simulink model "parts"  (R2021b)
settings: Solver=ode15s  StartTime=0.0  StopTime=t_f  MaxStep=max_step_size  RelTol=1e-3
values from neighbouring files (symbols this model uses):
  cont_param_10 = in    [double_pendulum.m]    (also in optimize_10_SMC_single_first_explicit.m = cont_param_10_surrogateopt)
  cont_param_11 = in    [double_pendulum.m]    (also in optimize_11_SMC_single_first_implicit.m = cont_param_11_surrogateopt)
  cont_param_12 = in    [double_pendulum.m]    (also in optimize_12_SMC_single_last_explicit.m = cont_param_12_surrogateopt)
  cont_param_13 = in    [double_pendulum.m]    (also in optimize_13_SMC_single_last_implicit.m = cont_param_13_surrogateopt)
  cont_param_14 = in    [double_pendulum.m]    (also in optimize_14_SMC_double_explicit.m = cont_param_14_surrogateopt)
  cont_param_15 = in    [double_pendulum.m]    (also in optimize_15_SMC_double_implicit.m = cont_param_15_surrogateopt)
  cont_param_16 = in    [double_pendulum.m]
  cont_param_17 = in    [double_pendulum.m]
  cont_param_18 = in    [double_pendulum.m]
  cont_param_19 = in    [double_pendulum.m]
  cont_param_4 = in    [double_pendulum.m]
  cont_param_5 = in    [double_pendulum.m]
  cont_param_6 = in    [double_pendulum.m]
  cont_param_7 = in    [double_pendulum.m]
  cont_param_8 = in    [double_pendulum.m]
  cont_param_9 = in    [double_pendulum.m]
  h = 1e-5    (= 1e-05)    [Conference_paper.m]    (also in Latest.m)
  m = 10    [Conference_paper.m]    (also in Latest.m = 100; control_8_collocated_PD_tracking.m = load_mass+hook_mass+cable_mass_total)
  method_select = Method    [main_run.m]    (also in modify_tracking.m = 3)
  N = floor(t_f / h)    [control_2_zero_vibration.m]    (also in control_3_ZVD.m; modify_tracking.m = 3)
  s = c1*(x-xd)+c2*(v-vd)+c3*theta_dot_1+c4*theta_1    [control_10_SMC_single_first_explicit.m]    (also in control_11_SMC_single_first_implicit.m = c1*(x-xd)+c2*(v-vd)+c3*theta_dot+c4*theta; control_12_SMC_single_last_explicit.m = c1*(x-xd)+c2*(v-vd)+c3*theta_dot_2+c4*theta_2; control_13_SMC_single_last_implicit.m = c1*(x-xd)+c2*(v-vd)+c3*theta_dot+c4*theta; control_14_SMC_double_explicit.m = (v-vd)+lambda*(x-xd)+alpha*theta_1+beta*theta_2)
  X = ex+lambda*sin(theta)    [control_16_PD_energy_first.m]    (also in control_17_PD_energy_last.m)
  Z = cont_param_8(4)    [control_8_collocated_PD_tracking.m]
undefined symbols (not defined in the file or in its folder): a_d_full, all_initial_sway, c_actuator, cable_eact_piece, cable_length, cable_mass_total, cart_disturbance_amp, cart_mass, delay_time, first_link_sway, hook_mass, last_piece_length, load_disturbance_amp, number_of_pendulums, payload_mass, sat_const, t_f, total_mass, traj_number, Y
libraries: sm_lib x72, nesl_utility x47, commchan3 x4
(part 2 of 2)

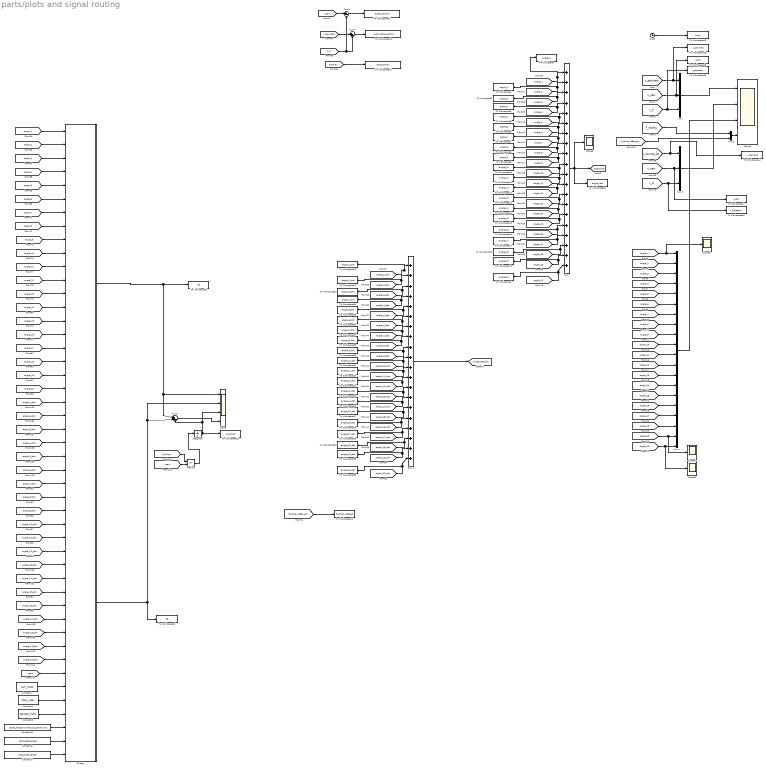
== system parts/plots and signal routing ==
  Clock : Clock
  Constant : Constant  Value=cart_mass
  Constant1 : Constant  Value=hook_mass
  Constant11 : Constant  Value=cable_length/number_of_pendulums
  Constant2 : Constant  Value=payload_mass
  Constant3 : Constant  Value=cable_eact_piece
  Constant4 : Constant  Value=last_piece_length
  Energy : MATLAB Function  TreatAsAtomicUnit=on
  Integrator : Integrator
  Mux : Mux  Inputs=3
  Mux1 : Mux  Inputs=20
  Mux2 : Mux  Inputs=3
  Mux3 : Mux  Inputs=2
  Product : Product
  Scope : Scope  NumInputPorts=4
  Scope1 : Scope  NumInputPorts=4
  Scope{3..6} (4 alike) : Scope
  Sum : Sum  Inputs=|++++++++++++++++++++
  Sum1 : Sum  Inputs=|++++++++++++++++++++
  Sum2 : Sum  Inputs=|+-
  Sum3 : Sum  Inputs=|+-
  Sum4 : Sum  Inputs=|++-
  To Workspace : ToWorkspace  VariableName=angle_1  SampleTime=-1
  To Workspace1 : ToWorkspace  VariableName=angle_2  SampleTime=-1
  To Workspace10 : ToWorkspace  VariableName=angle_10  SampleTime=-1
  To Workspace11 : ToWorkspace  VariableName=angle_11  SampleTime=-1
  To Workspace12 : ToWorkspace  VariableName=angle_12  SampleTime=-1
  To Workspace13 : ToWorkspace  VariableName=angle_13  SampleTime=-1
  To Workspace14 : ToWorkspace  VariableName=angle_14  SampleTime=-1
  To Workspace15 : ToWorkspace  VariableName=angle_15  SampleTime=-1
  To Workspace16 : ToWorkspace  VariableName=angle_16  SampleTime=-1
  To Workspace17 : ToWorkspace  VariableName=angle_17  SampleTime=-1
  To Workspace18 : ToWorkspace  VariableName=angle_18  SampleTime=-1
  To Workspace19 : ToWorkspace  VariableName=angle_19  SampleTime=-1
  To Workspace2 : ToWorkspace  VariableName=angle_3  SampleTime=-1
  To Workspace20 : ToWorkspace  VariableName=angle_1_dot  SampleTime=-1
  To Workspace21 : ToWorkspace  VariableName=angle_2_dot  SampleTime=-1
  To Workspace22 : ToWorkspace  VariableName=angle_10_dot  SampleTime=-1
  To Workspace23 : ToWorkspace  VariableName=angle_11_dot  SampleTime=-1
  To Workspace24 : ToWorkspace  VariableName=angle_12_dot  SampleTime=-1
  To Workspace25 : ToWorkspace  VariableName=angle_13_dot  SampleTime=-1
  To Workspace26 : ToWorkspace  VariableName=angle_14_dot  SampleTime=-1
  To Workspace27 : ToWorkspace  VariableName=angle_15_dot  SampleTime=-1
  To Workspace28 : ToWorkspace  VariableName=angle_16_dot  SampleTime=-1
  To Workspace29 : ToWorkspace  VariableName=angle_17_dot  SampleTime=-1
  To Workspace3 : ToWorkspace  VariableName=angle_20  SampleTime=-1
  To Workspace30 : ToWorkspace  VariableName=angle_18_dot  SampleTime=-1
  To Workspace31 : ToWorkspace  VariableName=angle_19_dot  SampleTime=-1
  To Workspace32 : ToWorkspace  VariableName=angle_3_dot  SampleTime=-1
  To Workspace33 : ToWorkspace  VariableName=angle_20_dot  SampleTime=-1
  To Workspace34 : ToWorkspace  VariableName=angle_4_dot  SampleTime=-1
  To Workspace35 : ToWorkspace  VariableName=angle_5_dot  SampleTime=-1
  To Workspace36 : ToWorkspace  VariableName=angle_6_dot  SampleTime=-1
  To Workspace37 : ToWorkspace  VariableName=angle_7_dot  SampleTime=-1
  To Workspace38 : ToWorkspace  VariableName=angle_8_dot  SampleTime=-1
  To Workspace39 : ToWorkspace  VariableName=angle_9_dot  SampleTime=-1
  To Workspace4 : ToWorkspace  VariableName=angle_4  SampleTime=-1
  To Workspace40 : ToWorkspace  VariableName=e_payload_position  SampleTime=-1
  To Workspace41 : ToWorkspace  VariableName=Force_trolley  SampleTime=-1
  To Workspace42 : ToWorkspace  VariableName=e_cart_position  SampleTime=-1
  To Workspace43 : ToWorkspace  VariableName=x_payload  SampleTime=-1
  To Workspace44 : ToWorkspace  VariableName=v_payload  SampleTime=-1
  To Workspace45 : ToWorkspace  VariableName=x_cart  SampleTime=-1
  To Workspace46 : ToWorkspace  VariableName=x_trajectory  SampleTime=-1
  To Workspace47 : ToWorkspace  VariableName=v_cart  SampleTime=-1
  To Workspace48 : ToWorkspace  VariableName=v_trajectory  SampleTime=-1
  To Workspace49 : ToWorkspace  VariableName=time  SampleTime=-1
  To Workspace5 : ToWorkspace  VariableName=angle_5  SampleTime=-1
  To Workspace50 : ToWorkspace  VariableName=angle_last  SampleTime=-1
  To Workspace51 : ToWorkspace  VariableName=KE  SampleTime=-1
  To Workspace52 : ToWorkspace  VariableName=PE  SampleTime=-1
  To Workspace53 : ToWorkspace  VariableName=supplied  SampleTime=-1
  To Workspace54 : ToWorkspace  VariableName=F_trolley_filtered  SampleTime=-1
  To Workspace6 : ToWorkspace  VariableName=angle_6  SampleTime=-1
  To Workspace7 : ToWorkspace  VariableName=angle_7  SampleTime=-1
  To Workspace8 : ToWorkspace  VariableName=angle_8  SampleTime=-1
  To Workspace9 : ToWorkspace  VariableName=angle_9  SampleTime=-1
  tag scope: angle_last=global, angle_last_dot=global
  wires:
  Mux/1 -> Scope1/1
  [x_payload] -> To Workspace43/1, Mux/1  "x_payload"
  [x_cart] -> To Workspace45/1, Mux/2  "x_cart"
  [x_d] -> To Workspace46/1, Mux/3  "x_trajectory"
  Mux1/1 -> Scope1/3
  [angle_1] -> Scope3/1, Mux1/1  "Angle 1"
  [angle_2] -> Mux1/2  "Angle 2"
  [angle_3] -> Mux1/3  "Angle 3"
  [angle_4] -> Mux1/4  "Angle 4"
  [angle_5] -> Mux1/5  "Angle 5"
  [angle_6] -> Mux1/6  "Angle 6"
  [angle_7] -> Mux1/7  "Angle 7"
  [angle_8] -> Mux1/8  "Angle 8"
  [angle_9] -> Mux1/9  "Angle 9"
  [angle_10] -> Mux1/10  "Angle 10"
  [angle_11] -> Mux1/11  "Angle 11"
  [angle_12] -> Mux1/12  "Angle 12"
  [angle_13] -> Mux1/13  "Angle 13"
  [angle_14] -> Mux1/14  "Angle 14"
  [angle_15] -> Mux1/15  "Angle 15"
  [angle_16] -> Mux1/16  "Angle 16"
  [angle_17] -> Mux1/17  "Angle 17"
  [angle_18] -> Mux1/18  "Angle 18"
  [angle_19] -> Scope4/1, Mux1/19  "Angle 19"
  [angle_1] -> To Workspace/1, Sum/1  "Angle 1"
  [angle_2] -> To Workspace1/1, Sum/2  "Angle 2"
  [angle_3] -> To Workspace2/1, Sum/3  "Angle 3"
  [angle_4] -> To Workspace4/1, Sum/4  "Angle 4"
  [angle_5] -> To Workspace5/1, Sum/5  "Angle 5"
  [angle_6] -> To Workspace6/1, Sum/6  "Angle 6"
  [angle_7] -> To Workspace7/1, Sum/7  "Angle 7"
  [angle_8] -> To Workspace8/1, Sum/8  "Angle 8"
  [angle_9] -> To Workspace9/1, Sum/9  "Angle 9"
  [angle_10] -> To Workspace10/1, Sum/10  "Angle 10"
  [angle_11] -> To Workspace11/1, Sum/11  "Angle 11"
  [angle_12] -> To Workspace12/1, Sum/12  "Angle 12"
  [angle_13] -> To Workspace13/1, Sum/13  "Angle 13"
  [angle_14] -> To Workspace14/1, Sum/14  "Angle 14"
  [angle_15] -> To Workspace15/1, Sum/15  "Angle 15"
  [angle_16] -> To Workspace16/1, Sum/16  "Angle 16"
  [angle_17] -> To Workspace17/1, Sum/17  "Angle 17"
  [angle_18] -> To Workspace18/1, Sum/18  "Angle 18"
  [angle_19] -> To Workspace19/1, Sum/19  "Angle 19"
  Sum/1 -> To Workspace50/1, Scope6/1, [angle_last]
  [angle_20] -> Scope5/1, Mux1/20  "Angle 20"
  [angle_20] -> To Workspace3/1, Sum/20  "Angle 19"
  [angle_6_dot] -> To Workspace36/1, Sum1/6  "Angle 6"
  [angle_19_dot] -> To Workspace31/1, Sum1/19  "Angle 19"
  [angle_3_dot] -> To Workspace32/1, Sum1/3  "Angle 3"
  [angle_17_dot] -> To Workspace29/1, Sum1/17  "Angle 17"
  Sum1/1 -> [angle_last_dot]
  [angle_16_dot] -> To Workspace28/1, Sum1/16  "Angle 16"
  [angle_18_dot] -> To Workspace30/1, Sum1/18  "Angle 18"
  [angle_10_dot] -> To Workspace22/1, Sum1/10  "Angle 10"
  [angle_5_dot] -> To Workspace35/1, Sum1/5  "Angle 5"
  [angle_2_dot] -> To Workspace21/1, Sum1/2  "Angle 2"
  [angle_11_dot] -> To Workspace23/1, Sum1/11  "Angle 11"
  [angle_1_dot] -> To Workspace20/1, Sum1/1  "Angle 1"
  [angle_4_dot] -> To Workspace34/1, Sum1/4  "Angle 4"
  [angle_15_dot] -> To Workspace27/1, Sum1/15  "Angle 15"
  [angle_7_dot] -> To Workspace37/1, Sum1/7  "Angle 7"
  [angle_12_dot] -> To Workspace24/1, Sum1/12  "Angle 12"
  [angle_14_dot] -> To Workspace26/1, Sum1/14  "Angle 14"
  [angle_13_dot] -> To Workspace25/1, Sum1/13  "Angle 13"
  [angle_20_dot] -> To Workspace33/1, Sum1/20  "Angle 19"
  [angle_9_dot] -> To Workspace39/1, Sum1/9  "Angle 9"
  [angle_8_dot] -> To Workspace38/1, Sum1/8  "Angle 8"
  Sum2/1 -> To Workspace40/1
  [F_trolley] -> To Workspace41/1
  [x_d] -> Sum3/2, Sum2/2
  [x_payload] -> Sum2/1
  [x_cart] -> Sum3/1
  Sum3/1 -> To Workspace42/1
  [v_cart] -> To Workspace47/1, Mux2/2  "v_cart"
  [v_d] -> To Workspace48/1, Mux2/3  "v_trajectory"
  [x_payload_dot] -> To Workspace44/1, Mux2/1  "v_payload"
  Mux2/1 -> Scope1/2
  Clock/1 -> To Workspace49/1
  [angle_1] -> Energy/1(theta1)  "Angle 1"
  [angle_2] -> Energy/2(theta2)  "Angle 2"
  [angle_3] -> Energy/3(theta3)  "Angle 3"
  [angle_4] -> Energy/4(theta4)  "Angle 4"
  [angle_5] -> Energy/5(theta5)  "Angle 5"
  [angle_6] -> Energy/6(theta6)  "Angle 6"
  [angle_7] -> Energy/7(theta7)  "Angle 7"
  [angle_8] -> Energy/8(theta8)  "Angle 8"
  [angle_9] -> Energy/9(theta9)  "Angle 9"
  [angle_10] -> Energy/10(theta10)  "Angle 10"
  [angle_11] -> Energy/11(theta11)  "Angle 11"
  [angle_12] -> Energy/12(theta12)  "Angle 12"
  [angle_13] -> Energy/13(theta13)  "Angle 13"
  [angle_14] -> Energy/14(theta14)  "Angle 14"
  [angle_15] -> Energy/15(theta15)  "Angle 15"
  [angle_16] -> Energy/16(theta16)  "Angle 16"
  [angle_17] -> Energy/17(theta17)  "Angle 17"
  [angle_18] -> Energy/18(theta18)  "Angle 18"
  [angle_19] -> Energy/19(theta19)  "Angle 19"
  [angle_20] -> Energy/20(theta20)  "Angle 20"
  [angle_1_dot] -> Energy/21(theta1_dot)  "Angle 1"
  [angle_2_dot] -> Energy/22(theta2_dot)  "Angle 2"
  [angle_3_dot] -> Energy/23(theta3_dot)  "Angle 3"
  [angle_4_dot] -> Energy/24(theta4_dot)  "Angle 4"
  [angle_5_dot] -> Energy/25(theta5_dot)  "Angle 5"
  [angle_6_dot] -> Energy/26(theta6_dot)  "Angle 6"
  [angle_7_dot] -> Energy/27(theta7_dot)  "Angle 7"
  [angle_8_dot] -> Energy/28(theta8_dot)  "Angle 8"
  [angle_9_dot] -> Energy/29(theta9_dot)  "Angle 9"
  [angle_10_dot] -> Energy/30(theta10_dot)  "Angle 10"
  [angle_11_dot] -> Energy/31(theta11_dot)  "Angle 11"
  [angle_12_dot] -> Energy/32(theta12_dot)  "Angle 12"
  [angle_13_dot] -> Energy/33(theta13_dot)  "Angle 13"
  [angle_14_dot] -> Energy/34(theta14_dot)  "Angle 14"
  [angle_15_dot] -> Energy/35(theta15_dot)  "Angle 15"
  [angle_16_dot] -> Energy/36(theta16_dot)  "Angle 16"
  [angle_17_dot] -> Energy/37(theta17_dot)  "Angle 17"
  [angle_18_dot] -> Energy/38(theta18_dot)  "Angle 18"
  [angle_19_dot] -> Energy/39(theta19_dot)  "Angle 19"
  [angle_20_dot] -> Energy/40(theta20_dot)  "Angle 19"
  [v_cart] -> Energy/41(v_cart)
  Constant/1 -> Energy/42(cart_mass)
  Constant1/1 -> Energy/43(hook_mass)
  Constant2/1 -> Energy/44(payload_mass)
  Constant11/1 -> Energy/45(piece_length)
  Constant3/1 -> Energy/46(piece_mass)
  Energy/1(KE) -> To Workspace51/1, Sum4/1, Scope/1  "KE"
  Energy/2(PE) -> To Workspace52/1, Sum4/2, Scope/2  "PE"
  [v_cart] -> Product/2  "Angle 17"
  Integrator/1 -> To Workspace53/1, Scope/3, Sum4/3  "Supplied energy"
  Product/1 -> Integrator/1
  [F_trolley] -> Product/1  "Angle 17"
  Sum4/1 -> Scope/4  "PE+KE-supply"
  Constant4/1 -> Energy/47(last_piece_length)
  [F_trolley_after_act] -> To Workspace54/1
  Mux3/1 -> Scope1/4
  [F_trolley] -> Mux3/1  "Force_trolley"
  [F_trolley_after_act] -> Mux3/2  "Force_trolley_filtered"

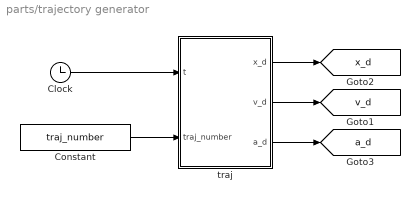
== system parts/trajectory generator ==
  Clock : Clock
  Constant : Constant  Value=traj_number
  traj : MATLAB Function  TreatAsAtomicUnit=on
  tag scope: a_d=global, v_d=global, x_d=global
  wires:
  traj/1(x_d) -> [x_d]
  Clock/1 -> traj/1(t)
  traj/2(v_d) -> [v_d]
  traj/3(a_d) -> [a_d]
  Constant/1 -> traj/2(traj_number)

== matlab function parts/trajectory generator/traj ==
  data: t input; x_d output; v_d output; a_d output; traj_number input
function [x_d,v_d,a_d] = traj_gen(t,traj_number)
     [x_d,v_d,a_d] = trajectory(t,traj_number);
end

== matlab function parts/plots and signal routing/Energy ==
  data: theta1 input; theta2 input; theta3 input; theta4 input; theta5 input; theta6 input; theta7 input; theta8 input; theta9 input; theta10 input; theta11 input; theta12 input; theta13 input; theta14 input; theta15 input; theta16 input; theta17 input; theta18 input; theta19 input; theta20 input; theta1_dot input; theta2_dot input; theta3_dot input; theta4_dot input; theta5_dot input; theta6_dot input; theta7_dot input; theta8_dot input; theta9_dot input; theta10_dot input; theta11_dot input; theta12_dot input; theta13_dot input; theta14_dot input; theta15_dot input; theta16_dot input; theta17_dot input; theta18_dot input; theta19_dot input; theta20_dot input; v_cart input; cart_mass input; hook_mass input; payload_mass input; piece_length input; piece_mass input; KE output; PE output; last_piece_length input
function [KE,PE]   = Energy_calc(theta1,theta2,theta3,theta4,theta5,theta6,theta7,theta8,theta9,theta10,theta11,theta12,theta13,theta14,theta15,theta16,theta17,theta18,theta19,theta20,theta1_dot,theta2_dot,theta3_dot,theta4_dot,theta5_dot,theta6_dot,theta7_dot,theta8_dot,theta9_dot,theta10_dot,theta11_dot,theta12_dot,theta13_dot,theta14_dot,theta15_dot,theta16_dot,theta17_dot,theta18_dot,theta19_dot,theta20_dot,v_cart,cart_mass,hook_mass,payload_mass,piece_length,piece_mass,last_piece_length)
     
    theta1=mod(theta1,2*pi);
    theta2=mod(theta2,2*pi);
    theta3=mod(theta3,2*pi);
    theta4=mod(theta4,2*pi);
    theta5=mod(theta5,2*pi);
    theta6=mod(theta6,2*pi);
    theta7=mod(theta7,2*pi);
    theta8=mod(theta8,2*pi);
    theta9=mod(theta9,2*pi);
    theta10=mod(theta10,2*pi);
    theta11=mod(theta11,2*pi);
    theta12=mod(theta12,2*pi);
    theta13=mod(theta13,2*pi);
    theta14=mod(theta14,2*pi);
    theta15=mod(theta15,2*pi);
    theta16=mod(theta16,2*pi);
    theta17=mod(theta17,2*pi);
    theta18=mod(theta18,2*pi);
    theta19=mod(theta19,2*pi);
    theta20=mod(theta20,2*pi);



    l=piece_length;
    g=9.8;
    
    y1=-l*cos(theta1);
    y2=-l*cos(theta1+theta2)+y1;
    y3=-l*cos(theta1+theta2+theta3)+y2;
    y4=-l*cos(theta1+theta2+theta3+theta4)+y3;
    y5=-l*cos(theta1+theta2+theta3+theta4+theta5)+y4;
    y6=-l*cos(theta1+theta2+theta3+theta4+theta5+theta6)+y5;
    y7=-l*cos(theta1+theta2+theta3+theta4+theta5+theta6+theta7)+y6;
    y8=-l*cos(theta1+theta2+theta3+theta4+theta5+theta6+theta7+theta8)+y7;
    y9=-l*cos(theta1+theta2+theta3+theta4+theta5+theta6+theta7+theta8+theta9)+y8;
    y10=-l*cos(theta1+theta2+theta3+theta4+theta5+theta6+theta7+theta8+theta9+theta10)+y9;
    y11=-l*cos(theta1+theta2+theta3+theta4+theta5+theta6+theta7+theta8+theta9+theta10+theta11)+y10;
    y12=-l*cos(theta1+theta2+theta3+theta4+theta5+theta6+theta7+theta8+theta9+theta10+theta11+theta12)+y11;
    y13=-l*cos(theta1+theta2+theta3+theta4+theta5+theta6+theta7+theta8+theta9+theta10+theta11+theta12+theta13)+y12;
    y14=-l*cos(theta1+theta2+theta3+theta4+theta5+theta6+theta7+theta8+theta9+theta10+theta11+theta12+theta13+theta14)+y13;
    y15=-l*cos(theta1+theta2+theta3+theta4+theta5+theta6+theta7+theta8+theta9+theta10+theta11+theta12+theta13+theta14+theta15)+y14;
    y16=-l*cos(theta1+theta2+theta3+theta4+theta5+theta6+theta7+theta8+theta9+theta10+theta11+theta12+theta13+theta14+theta15+theta16)+y15;
    y17=-l*cos(theta1+theta2+theta3+theta4+theta5+theta6+theta7+theta8+theta9+theta10+theta11+theta12+theta13+theta14+theta15+theta16+theta17)+y16;
    y18=-l*cos(theta1+theta2+theta3+theta4+theta5+theta6+theta7+theta8+theta9+theta10+theta11+theta12+theta13+theta14+theta15+theta16+theta17+theta18)+y17;
    y19=-l*cos(theta1+theta2+theta3+theta4+theta5+theta6+theta7+theta8+theta9+theta10+theta11+theta12+theta13+theta14+theta15+theta16+theta17+theta18+theta19)+y18;
    y20=-last_piece_length*cos(theta1+theta2+theta3+theta4+theta5+theta6+theta7+theta8+theta9+theta10+theta11+theta12+theta13+theta14+theta15+theta16+theta17+theta18+theta19+theta20)+y19;
    
    
    
    
    
    x_dot1=l*cos(theta1)*theta1_dot+v_cart;
    x_dot2=l*cos(theta1+theta2)*(theta1_dot+theta2_dot)+x_dot1;
    x_dot3=l*cos(theta1+theta2+theta3)*(theta1_dot+theta2_dot+theta3_dot)+x_dot2;
    x_dot4=l*cos(theta1+theta2+theta3+theta4)*(theta1_dot+theta2_dot+theta3_dot+theta4_dot)+x_dot3;
    x_dot5=l*cos(theta1+theta2+theta3+theta4+theta5)*(theta1_dot+theta2_dot+theta3_dot+theta4_dot+theta5_dot)+x_dot4;
    x_dot6=l*cos(theta1+theta2+theta3+theta4+theta5+theta6)*(theta1_dot+theta2_dot+theta3_dot+theta4_dot+theta5_dot+theta6_dot)+x_dot5;
    x_dot7=l*cos(theta1+theta2+theta3+theta4+theta5+theta6+theta7)*(theta1_dot+theta2_dot+theta3_dot+theta4_dot+theta5_dot+theta6_dot+theta7_dot)+x_dot6;
    x_dot8=l*cos(theta1+theta2+theta3+theta4+theta5+theta6+theta7+theta8)*(theta1_dot+theta2_dot+theta3_dot+theta4_dot+theta5_dot+theta6_dot+theta7_dot+theta8_dot)+x_dot7;
    x_dot9=l*cos(theta1+theta2+theta3+theta4+theta5+theta6+theta7+theta8+theta9)*(theta1_dot+theta2_dot+theta3_dot+theta4_dot+theta5_dot+theta6_dot+theta7_dot+theta8_dot+theta9_dot)+x_dot8;
    x_dot10=l*cos(theta1+theta2+theta3+theta4+theta5+theta6+theta7+theta8+theta9+theta10)*(theta1_dot+theta2_dot+theta3_dot+theta4_dot+theta5_dot+theta6_dot+theta7_dot+theta8_dot+theta9_dot+theta10_dot)+x_dot9;
    x_dot11=l*cos(theta1+theta2+theta3+theta4+theta5+theta6+theta7+theta8+theta9+theta10+theta11)*(theta1_dot+theta2_dot+theta3_dot+theta4_dot+theta5_dot+theta6_dot+theta7_dot+theta8_dot+theta9_dot+theta10_dot+theta11_dot)+x_dot10;
    x_dot12=l*cos(theta1+theta2+theta3+theta4+theta5+theta6+theta7+theta8+theta9+theta10+theta11+theta12)*(theta1_dot+theta2_dot+theta3_dot+theta4_dot+theta5_dot+theta6_dot+theta7_dot+theta8_dot+theta9_dot+theta10_dot+theta11_dot+theta12_dot)+x_dot11;
    x_dot13=l*cos(theta1+theta2+theta3+theta4+theta5+theta6+theta7+theta8+theta9+theta10+theta11+theta12+theta13)*(theta1_dot+theta2_dot+theta3_dot+theta4_dot+theta5_dot+theta6_dot+theta7_dot+theta8_dot+theta9_dot+theta10_dot+theta11_dot+theta12_dot+theta13_dot)+x_dot12;
    x_dot14=l*cos(theta1+theta2+theta3+theta4+theta5+theta6+theta7+theta8+theta9+theta10+theta11+theta12+theta13+theta14)*(theta1_dot+theta2_dot+theta3_dot+theta4_dot+theta5_dot+theta6_dot+theta7_dot+theta8_dot+theta9_dot+theta10_dot+theta11_dot+theta12_dot+theta13_dot+theta14_dot)+x_dot13;
    x_dot15=l*cos(theta1+theta2+theta3+theta4+theta5+theta6+theta7+theta8+theta9+theta10+theta11+theta12+theta13+theta14+theta15)*(theta1_dot+theta2_dot+theta3_dot+theta4_dot+theta5_dot+theta6_dot+theta7_dot+theta8_dot+theta9_dot+theta10_dot+theta11_dot+theta12_dot+theta13_dot+theta14_dot+theta15_dot)+x_dot14;
    x_dot16=l*cos(theta1+theta2+theta3+theta4+theta5+theta6+theta7+theta8+theta9+theta10+theta11+theta12+theta13+theta14+theta15+theta16)*(theta1_dot+theta2_dot+theta3_dot+theta4_dot+theta5_dot+theta6_dot+theta7_dot+theta8_dot+theta9_dot+theta10_dot+theta11_dot+theta12_dot+theta13_dot+theta14_dot+theta15_dot+theta16_dot)+x_dot15;
    x_dot17=l*cos(theta1+theta2+theta3+theta4+theta5+theta6+theta7+theta8+theta9+theta10+theta11+theta12+theta13+theta14+theta15+theta16+theta17)*(theta1_dot+theta2_dot+theta3_dot+theta4_dot+theta5_dot+theta6_dot+theta7_dot+theta8_dot+theta9_dot+theta10_dot+theta11_dot+theta12_dot+theta13_dot+theta14_dot+theta15_dot+theta16_dot+theta17_dot)+x_dot16;
    x_dot18=l*cos(theta1+theta2+theta3+theta4+theta5+theta6+theta7+theta8+theta9+theta10+theta11+theta12+theta13+theta14+theta15+theta16+theta17+theta18)*(theta1_dot+theta2_dot+theta3_dot+theta4_dot+theta5_dot+theta6_dot+theta7_dot+theta8_dot+theta9_dot+theta10_dot+theta11_dot+theta12_dot+theta13_dot+theta14_dot+theta15_dot+theta16_dot+theta17_dot+theta18_dot)+x_dot17;
    x_dot19=cos(theta1+theta2+theta3+theta4+theta5+theta6+theta7+theta8+theta9+theta10+theta11+theta12+theta13+theta14+theta15+theta16+theta17+theta18+theta19)*(theta1_dot+theta2_dot+theta3_dot+theta4_dot+theta5_dot+theta6_dot+theta7_dot+theta8_dot+theta9_dot+theta10_dot+theta11_dot+theta12_dot+theta13_dot+theta14_dot+theta15_dot+theta16_dot+theta17_dot+theta18_dot+theta19_dot)+x_dot18;
    x_dot20=cos(theta1+theta2+theta3+theta4+theta5+theta6+theta7+theta8+theta9+theta10+theta11+theta12+theta13+theta14+theta15+theta16+theta17+theta18+theta19+theta20)*(theta1_dot+theta2_dot+theta3_dot+theta4_dot+theta5_dot+theta6_dot+theta7_dot+theta8_dot+theta9_dot+theta10_dot+theta11_dot+theta12_dot+theta13_dot+theta14_dot+theta15_dot+theta16_dot+theta17_dot+theta18_dot+theta19_dot+theta20_dot)+x_dot19;
    
    y_dot1=-l*sin(theta1)*theta1_dot;
    y_dot2=-l*sin(theta1+theta2)*(theta1_dot+theta2_dot)+y_dot1;
    y_dot3=-l*sin(theta1+theta2+theta3)*(theta1_dot+theta2_dot+theta3_dot)+y_dot2;
    y_dot4=-l*sin(theta1+theta2+theta3+theta4)*(theta1_dot+theta2_dot+theta3_dot+theta4_dot)+y_dot3;
    y_dot5=-l*sin(theta1+theta2+theta3+theta4+theta5)*(theta1_dot+theta2_dot+theta3_dot+theta4_dot+theta5_dot)+y_dot4;
    y_dot6=-l*sin(theta1+theta2+theta3+theta4+theta5+theta6)*(theta1_dot+theta2_dot+theta3_dot+theta4_dot+theta5_dot+theta6_dot)+y_dot5;
    y_dot7=-l*sin(theta1+theta2+theta3+theta4+theta5+theta6+theta7)*(theta1_dot+theta2_dot+theta3_dot+theta4_dot+theta5_dot+theta6_dot+theta7_dot)+y_dot6;
    y_dot8=-l*sin(theta1+theta2+theta3+theta4+theta5+theta6+theta7+theta8)*(theta1_dot+theta2_dot+theta3_dot+theta4_dot+theta5_dot+theta6_dot+theta7_dot+theta8_dot)+y_dot7;
    y_dot9=-l*sin(theta1+theta2+theta3+theta4+theta5+theta6+theta7+theta8+theta9)*(theta1_dot+theta2_dot+theta3_dot+theta4_dot+theta5_dot+theta6_dot+theta7_dot+theta8_dot+theta9_dot)+y_dot8;
    y_dot10=-l*sin(theta1+theta2+theta3+theta4+theta5+theta6+theta7+theta8+theta9+theta10)*(theta1_dot+theta2_dot+theta3_dot+theta4_dot+theta5_dot+theta6_dot+theta7_dot+theta8_dot+theta9_dot+theta10_dot)+y_dot9;
    y_dot11=-l*sin(theta1+theta2+theta3+theta4+theta5+theta6+theta7+theta8+theta9+theta10+theta11)*(theta1_dot+theta2_dot+theta3_dot+theta4_dot+theta5_dot+theta6_dot+theta7_dot+theta8_dot+theta9_dot+theta10_dot+theta11_dot)+y_dot10;
    y_dot12=-l*sin(theta1+theta2+theta3+theta4+theta5+theta6+theta7+theta8+theta9+theta10+theta11+theta12)*(theta1_dot+theta2_dot+theta3_dot+theta4_dot+theta5_dot+theta6_dot+theta7_dot+theta8_dot+theta9_dot+theta10_dot+theta11_dot+theta12_dot)+y_dot11;
    y_dot13=-l*sin(theta1+theta2+theta3+theta4+theta5+theta6+theta7+theta8+theta9+theta10+theta11+theta12+theta13)*(theta1_dot+theta2_dot+theta3_dot+theta4_dot+theta5_dot+theta6_dot+theta7_dot+theta8_dot+theta9_dot+theta10_dot+theta11_dot+theta12_dot+theta13_dot)+y_dot12;
    y_dot14=-l*sin(theta1+theta2+theta3+theta4+theta5+theta6+theta7+theta8+theta9+theta10+theta11+theta12+theta13+theta14)*(theta1_dot+theta2_dot+theta3_dot+theta4_dot+theta5_dot+theta6_dot+theta7_dot+theta8_dot+theta9_dot+theta10_dot+theta11_dot+theta12_dot+theta13_dot+theta14_dot)+y_dot13;
    y_dot15=-l*sin(theta1+theta2+theta3+theta4+theta5+theta6+theta7+theta8+theta9+theta10+theta11+theta12+theta13+theta14+theta15)*(theta1_dot+theta2_dot+theta3_dot+theta4_dot+theta5_dot+theta6_dot+theta7_dot+theta8_dot+theta9_dot+theta10_dot+theta11_dot+theta12_dot+theta13_dot+theta14_dot+theta15_dot)+y_dot14;
    y_dot16=-l*sin(theta1+theta2+theta3+theta4+theta5+theta6+theta7+theta8+theta9+theta10+theta11+theta12+theta13+theta14+theta15+theta16)*(theta1_dot+theta2_dot+theta3_dot+theta4_dot+theta5_dot+theta6_dot+theta7_dot+theta8_dot+theta9_dot+theta10_dot+theta11_dot+theta12_dot+theta13_dot+theta14_dot+theta15_dot+theta16_dot)+y_dot15;
    y_dot17=-l*sin(theta1+theta2+theta3+theta4+theta5+theta6+theta7+theta8+theta9+theta10+theta11+theta12+theta13+theta14+theta15+theta16+theta17)*(theta1_dot+theta2_dot+theta3_dot+theta4_dot+theta5_dot+theta6_dot+theta7_dot+theta8_dot+theta9_dot+theta10_dot+theta11_dot+theta12_dot+theta13_dot+theta14_dot+theta15_dot+theta16_dot+theta17_dot)+y_dot16;
    y_dot18=-l*sin(theta1+theta2+theta3+theta4+theta5+theta6+theta7+theta8+theta9+theta10+theta11+theta12+theta13+theta14+theta15+theta16+theta17+theta18)*(theta1_dot+theta2_dot+theta3_dot+theta4_dot+theta5_dot+theta6_dot+theta7_dot+theta8_dot+theta9_dot+theta10_dot+theta11_dot+theta12_dot+theta13_dot+theta14_dot+theta15_dot+theta16_dot+theta17_dot+theta18_dot)+y_dot17;
    y_dot19=-sin(theta1+theta2+theta3+theta4+theta5+theta6+theta7+theta8+theta9+theta10+theta11+theta12+theta13+theta14+theta15+theta16+theta17+theta18+theta19)*(theta1_dot+theta2_dot+theta3_dot+theta4_dot+theta5_dot+theta6_dot+theta7_dot+theta8_dot+theta9_dot+theta10_dot+theta11_dot+theta12_dot+theta13_dot+theta14_dot+theta15_dot+theta16_dot+theta17_dot+theta18_dot+theta19_dot)+y_dot18;
    y_dot20=-sin(theta1+theta2+theta3+theta4+theta5+theta6+theta7+theta8+theta9+theta10+theta11+theta12+theta13+theta14+theta15+theta16+theta17+theta18+theta19+theta20)*(theta1_dot+theta2_dot+theta3_dot+theta4_dot+theta5_dot+theta6_dot+theta7_dot+theta8_dot+theta9_dot+theta10_dot+theta11_dot+theta12_dot+theta13_dot+theta14_dot+theta15_dot+theta16_dot+theta17_dot+theta18_dot+theta19_dot+theta20_dot)+y_dot19;
    
    
    KE0=0.5*cart_mass*(v_cart)^2;
    KE1=0.5*piece_mass*((x_dot1)^2+(y_dot1)^2);
    KE2=0.5*piece_mass*((x_dot2)^2+(y_dot2)^2);
    KE3=0.5*piece_mass*((x_dot3)^2+(y_dot3)^2);
    KE4=0.5*piece_mass*((x_dot4)^2+(y_dot4)^2);
    KE5=0.5*piece_mass*((x_dot5)^2+(y_dot5)^2);
    KE6=0.5*piece_mass*((x_dot6)^2+(y_dot6)^2);
    KE7=0.5*piece_mass*((x_dot7)^2+(y_dot7)^2);
    KE8=0.5*piece_mass*((x_dot8)^2+(y_dot8)^2);
    KE9=0.5*piece_mass*((x_dot9)^2+(y_dot9)^2);
    KE10=0.5*piece_mass*((x_dot10)^2+(y_dot10)^2);
    KE11=0.5*piece_mass*((x_dot11)^2+(y_dot11)^2);
    KE12=0.5*piece_mass*((x_dot12)^2+(y_dot12)^2);
    KE13=0.5*piece_mass*((x_dot13)^2+(y_dot13)^2);
    KE14=0.5*piece_mass*((x_dot14)^2+(y_dot14)^2);
    KE15=0.5*piece_mass*((x_dot15)^2+(y_dot15)^2);
    KE16=0.5*piece_mass*((x_dot16)^2+(y_dot16)^2);
    KE17=0.5*piece_mass*((x_dot17)^2+(y_dot17)^2);
    KE18=0.5*piece_mass*((x_dot18)^2+(y_dot18)^2);
    KE19=0.5*hook_mass*((x_dot19)^2+(y_dot19)^2);
    KE20=0.5*payload_mass*((x_dot20)^2+(y_dot20)^2);
    
    PE1=piece_mass*g*y1;
    PE2=piece_mass*g*y2;
    PE3=piece_mass*g*y3;
    PE4=piece_mass*g*y4;
    PE5=piece_mass*g*y5;
    PE6=piece_mass*g*y6;
    PE7=piece_mass*g*y7;
    PE8=piece_mass*g*y8;
    PE9=piece_mass*g*y9;
    PE10=piece_mass*g*y10;
    PE11=piece_mass*g*y11;
    PE12=piece_mass*g*y12;
    PE13=piece_mass*g*y13;
    PE14=piece_mass*g*y14;
    PE15=piece_mass*g*y15;
    PE16=piece_mass*g*y16;
    PE17=piece_mass*g*y17;
    PE18=piece_mass*g*y18;
    PE19=hook_mass*g*y19;
    PE20=payload_mass*g*y20;
    
    KE=KE0+KE1+KE2+KE3+KE4+KE5+KE6+KE7+KE8+KE9+KE10+KE11+KE12+KE13+KE14+KE15+KE16+KE17+KE18+KE19+KE20;
    PE=PE1+PE2+PE3+PE4+PE5+PE6+PE7+PE8+PE9+PE10+PE11+PE12+PE13+PE14+PE15+PE16+PE17+PE18+PE19+PE20;
    

end

== matlab function parts/controllers/Controllers ==
  data: x input; xd input; v input; vd input; theta_1 input; theta_2 input; theta1_dot input; theta2_dot input; trolley_mass input; hook_mass input; total_mass input; a_d input; a_d_full input; h input; t_f input; t input; cont_param_4 input; cont_param_5 input; cont_param_6 input; cont_param_7 input; cont_param_8 input; cont_param_9 input; cont_param_10 input; cont_param_11 input; cont_param_12 input; cont_param_13 input; cont_param_14 input; cont_param_15 input; cont_param_16 input; cont_param_17 input; cont_param_18 input; cont_param_19 input; cont_select input; cart_mass input; payload_mass input; cable_mass_total input; F output; cable_length input; last_piece_length input; counter_stopping_loop_in input; counter_stopping_loop output; run_flag output; run_flag_in input; break_signal output; break_signal_in input; cont_stop_time output; cont_stop_time_in input
function [F,counter_stopping_loop,run_flag,break_signal,cont_stop_time] = Control_select(x,xd,v,vd,theta_1,theta_2,theta1_dot,theta2_dot,trolley_mass,hook_mass,total_mass,a_d,a_d_full,h,t_f,t,cont_param_4,cont_param_5,cont_param_6,cont_param_7,cont_param_8,cont_param_9,cont_param_10,cont_param_11,cont_param_12,cont_param_13,cont_param_14,cont_param_15,cont_param_16,cont_param_17,cont_param_18,cont_param_19,cont_select,cart_mass,payload_mass,cable_mass_total,cable_length,last_piece_length,counter_stopping_loop_in,run_flag_in,break_signal_in,cont_stop_time_in)

    cont_stop_time=cont_stop_time_in;
    break_signal=break_signal_in;
    run_flag=run_flag_in;
    counter_stopping_loop=counter_stopping_loop_in;

    F = run_flag*Controllers(x,xd,v,vd,theta_1,theta_2,theta1_dot,theta2_dot,trolley_mass,hook_mass,total_mass,a_d,a_d_full,h,t_f,t,cont_param_4,cont_param_5,cont_param_6,cont_param_7,cont_param_8,cont_param_9,cont_param_10,cont_param_11,cont_param_12,cont_param_13,cont_param_14,cont_param_15,cont_param_16,cont_param_17,cont_param_18,cont_param_19,cont_select,cart_mass,payload_mass,cable_mass_total,cable_length,last_piece_length);
                 
    if isnan(F)
        F=0;
    end
    
    if abs(x-xd)<0.1 && abs(v)<0.02*3.5 && abs(theta_1)+abs(theta_2)<0.1*pi/180
        counter_stopping_loop=counter_stopping_loop+1;
    else
         counter_stopping_loop=0;
    end
    
    if counter_stopping_loop*h>8
        run_flag=0;
        break_signal=-1e6;
        cont_stop_time=t;
    end
        
    
end
